simulink model "untitled"  (R2013a)
settings: Solver=ode45  StartTime=0.0  StopTime=0.03  RelTol=1e-3
settings Model: Creator=Sion  LastModifiedBy=Sion

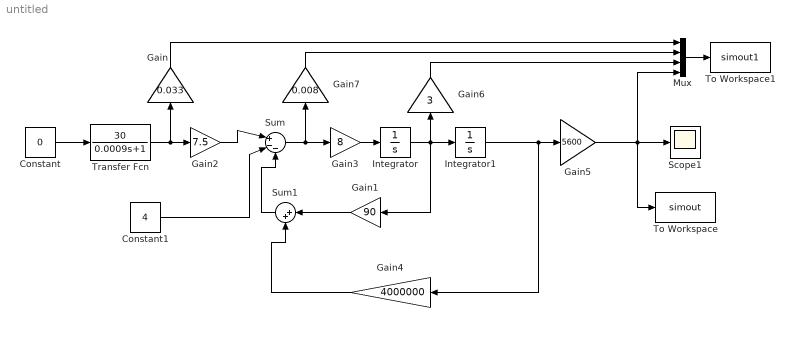
== system untitled ==
  Constant : Constant  Value=0
  Constant1 : Constant  Value=4
  Gain : Gain  Gain=0.033
  Gain1 : Gain  Gain=90
  Gain2 : Gain  Gain=7.5
  Gain3 : Gain  Gain=8
  Gain4 : Gain  Gain=4000000
  Gain5 : Gain  Gain=5600
  Gain6 : Gain  Gain=3
  Gain7 : Gain  Gain=0.008
  Integrator : Integrator
  Integrator1 : Integrator
  Mux : Mux
  Scope1 : Scope
      settings: SaveName=ScopeData3
  Sum : Sum  Inputs=|+--
  Sum1 : Sum  Inputs=|++
  To Workspace : ToWorkspace  VariableName=simout  SampleTime=-1  SaveFormat=Timeseries
  To Workspace1 : ToWorkspace  VariableName=simout1  SampleTime=-1  SaveFormat=Timeseries
  Transfer Fcn : TransferFcn  Numerator=[30]  Denominator=[0.0009 1]
  wires:
  Constant/1 -> Transfer Fcn/1
  Transfer Fcn/1 -> Gain2/1, Gain/1
  Gain4/1 -> Sum1/2
  Sum/1 -> Gain7/1, Gain3/1
  Gain2/1 -> Sum/1
  Gain3/1 -> Integrator/1
  Integrator/1 -> Integrator1/1, Gain1/1, Gain6/1
  Integrator1/1 -> Gain5/1, Gain4/1
  Gain1/1 -> Sum1/1
  Sum1/1 -> Sum/3
  Constant1/1 -> Sum/2
  Gain6/1 -> Mux/3
  Gain5/1 -> To Workspace/1, Scope1/1, Mux/4
  Mux/1 -> To Workspace1/1
  Gain7/1 -> Mux/2
  Gain/1 -> Mux/1
